simulink model "Doble_Pendulo"  (R2024a)
settings: Solver=VariableStepAuto  StartTime=0.0  StopTime=10  MaxStep=0.02  RelTol=1e-3
undefined symbols (not defined in the file): g, l1, l2, m1, m2
settings Model: Creator=mluser  LastModifiedBy=vicrr
settings OptimizationCC: ReuseModelBlockBuffer=off
settings RTWCC: GPUComputeCapability=3.5

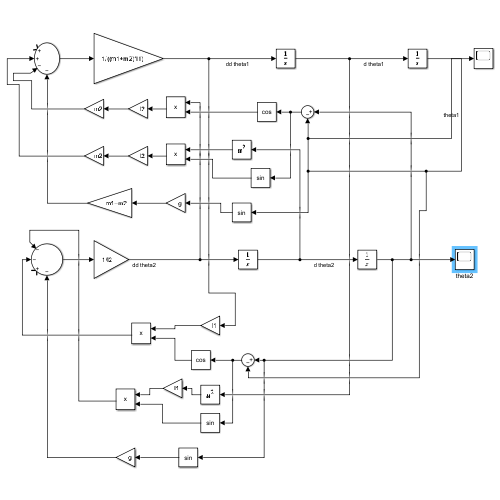
[thumbnail: Simulink's stored preview of the top-level diagram]
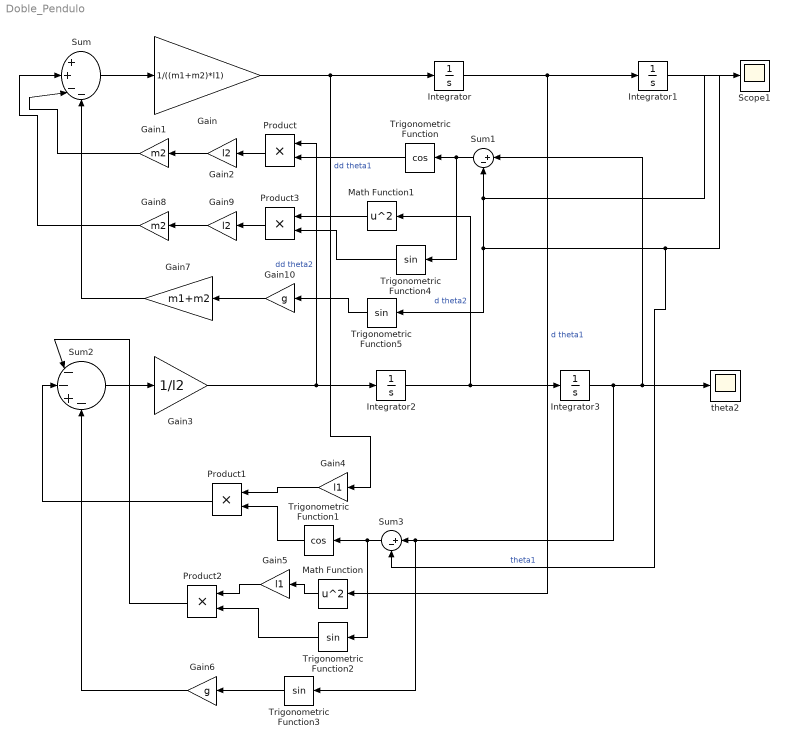
== system Doble_Pendulo ==
  Gain : Gain  Gain=1/((m1+m2)*l1)
  Gain1 : Gain  Gain=m2
  Gain10 : Gain  Gain=g
  Gain2 : Gain  Gain=l2
  Gain3 : Gain  Gain=1/l2
  Gain4 : Gain  Gain=l1
  Gain5 : Gain  Gain=l1
  Gain6 : Gain  Gain=g
  Gain7 : Gain  Gain=m1+m2
  Gain8 : Gain  Gain=m2
  Gain9 : Gain  Gain=l2
  Integrator : Integrator
  Integrator1 : Integrator
  Integrator2 : Integrator
  Integrator3 : Integrator  InitialCondition=(35*pi)/180
  Math Function : Math  Operator=square
  Math Function1 : Math  Operator=square
  Product{,1..3} (4 alike) : Product
  Scope1 : Scope
  Sum : Sum  Inputs=|++--
  Sum1 : Sum  Inputs=|+-
  Sum2 : Sum  Inputs=|--+-
  Sum3 : Sum  Inputs=|+-
  Trigonometric Function : Trigonometry  Operator=cos
  Trigonometric Function1 : Trigonometry  Operator=cos
  Trigonometric Function{2..5} (4 alike) : Trigonometry
  theta2 : Scope
  wires:
  Integrator/1 -> Math Function/1, Integrator1/1  "d theta1"
  Gain/1 -> Gain4/1, Integrator/1  "dd theta1"
  Sum/1 -> Gain/1
  Trigonometric Function/1 -> Product/2
  Sum1/1 -> Trigonometric Function/1, Trigonometric Function4/1
  Integrator1/1 -> Sum3/2, Trigonometric Function5/1, Sum1/2, Scope1/1  "theta1"
  Sum2/1 -> Gain3/1
  Gain3/1 -> Product/1, Integrator2/1  "dd theta2"
  Integrator2/1 -> Math Function1/1, Integrator3/1  "d theta2"
  Gain4/1 -> Product1/1
  Sum3/1 -> Trigonometric Function2/1, Trigonometric Function1/1
  Trigonometric Function1/1 -> Product1/2
  Integrator3/1 -> theta2/1, Sum1/1, Trigonometric Function3/1, Sum3/1
  Product1/1 -> Sum2/2
  Trigonometric Function2/1 -> Product2/2
  Math Function/1 -> Gain5/1
  Gain5/1 -> Product2/1
  Product2/1 -> Sum2/1
  Gain6/1 -> Sum2/4
  Trigonometric Function3/1 -> Gain6/1
  Gain2/1 -> Gain1/1
  Product/1 -> Gain2/1
  Gain1/1 -> Sum/3
  Trigonometric Function4/1 -> Product3/2
  Math Function1/1 -> Product3/1
  Gain8/1 -> Sum/2
  Product3/1 -> Gain9/1
  Gain9/1 -> Gain8/1
  Gain7/1 -> Sum/4
  Gain10/1 -> Gain7/1
  Trigonometric Function5/1 -> Gain10/1
